simulink model "CM660A_HwTq1Meas"  (R2013b)
settings: Solver=FixedStepDiscrete  StartTime=0.0  StopTime=20  FixedStep=0.002  RelTol=1e-3
values from neighbouring files (symbols this model uses):
  ELECGLBPRM_HWTQOFFS_HWNWTMTR_F32 = DataDict.Constant    [CM660A_HwTq1Meas_DataDict.m]
  ELECGLBPRM_HWTQSATNLOWRLIM_HWNWTMTR_F32 = DataDict.Constant    [CM660A_HwTq1Meas_DataDict.m]
  ELECGLBPRM_HWTQSATNUPPRLIM_HWNWTMTR_F32 = DataDict.Constant    [CM660A_HwTq1Meas_DataDict.m]
  ELECGLBPRM_HWTQSCA_ULS_F32 = DataDict.Constant    [CM660A_HwTq1Meas_DataDict.m]
  ELECGLBPRM_NOFLT_CNT_U08 = DataDict.Constant    [CM660A_HwTq1Meas_DataDict.m]
  ELECGLBPRM_OFFSTRIMNOTPRFM_CNT_U08 = DataDict.Constant    [CM660A_HwTq1Meas_DataDict.m]
  ELECGLBPRM_PRTCLFLT_CNT_U08 = DataDict.Constant    [CM660A_HwTq1Meas_DataDict.m]
  ELECGLBPRM_SNSRINTFLT_CNT_U08 = DataDict.Constant    [CM660A_HwTq1Meas_DataDict.m]
  HwTq1MeasHwTq1PrtclFltFailStep = DataDict.Calibration    [CM660A_HwTq1Meas_DataDict.m]
  HwTq1MeasHwTq1PrtclFltPassStep = DataDict.Calibration    [CM660A_HwTq1Meas_DataDict.m]
  RACKLIMRCCWEOTSCA_ULS_F32 = DataDict.Constant    [CM660A_HwTq1Meas_DataDict.m]
  RACKLIMRCWEOTSCA_ULS_F32 = DataDict.Constant    [CM660A_HwTq1Meas_DataDict.m]
undefined symbols (not defined in the file or in its folder): NtcNr1, NtcSts1, sigbuilder_block, SigQlfr1
libraries: simulink x25, NxtrNvM x3, NxtrLim x2
(part 2 of 3)

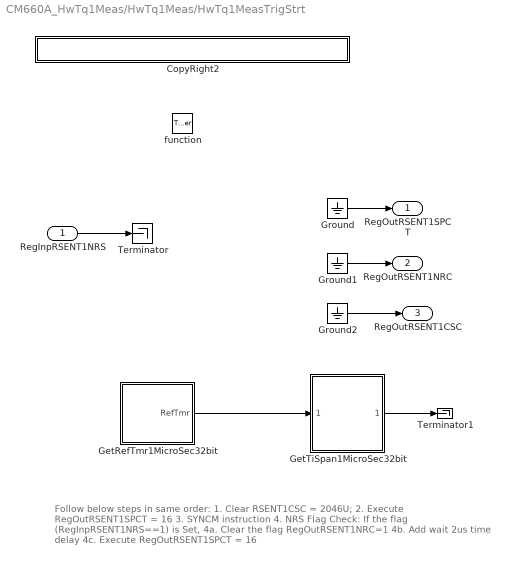
== system CM660A_HwTq1Meas/HwTq1Meas/HwTq1MeasTrigStrt ==
  note: Follow below steps in same order:
      |
      | 1. Clear RSENT1CSC = 2046U;
      | 2. Execute RegOutRSENT1SPCT = 16
      | 3. SYNCM instruction
      |
      | 4. NRS Flag Check: If the flag (RegInpRSENT1NRS==1) is Set,
      | 	4a. Clear the flag RegOutRSENT1NRC=1
      | 	4b. Add wait 2us time delay
      | 	4c. Execute RegOutRSENT1SPCT = 16
  RegInpRSENT1NRS : Inport
  function : TriggerPort  TriggerType=function-call
  CopyRight2 : Subsystem  Description=|  mask(Copyright Information){none=on}
      | Copyright info block.                                               
      |                                                                     
      | Place copyright information at the top of every subsystem in design.
      mask prompts: none "No parameters"
      mask help: Place copyright information at the top of every subsystem in design.
      mask Display:
      | NxtrConf = 'Nexteer Confidential';
      | 
      | sys = bdroot; %handle for the current model ("system")
      | first = get_param(sys,'Created');
      | first = first(end-3:end);  %year is last four digits
      | 
      | last = get_param(sys,'LastModifiedDate');
      | if isempty(last)
      |     last = datestr(now,'yyyy');
      | else
      |     last = last(end-3:end);
      | end
      | 
      | if strcmp(first,last)
      |     fprintf('%s -- Copyright %s Nexteer',NxtrConf,first)
      | else
      |     fprintf('%s -- %s%s- %s Nexteer',NxtrConf,char(169),first,last)
      | end
  GetRefTmr1MicroSec32bit : Subsystem
      settings: AttributesFormatString=Client Call : Start Time
  GetTiSpan1MicroSec32bit : Subsystem
  Ground : Ground
  Ground1 : Ground
  Ground2 : Ground
  Terminator : Terminator
  Terminator1 : Terminator
  RegOutRSENT1SPCT : Outport
  RegOutRSENT1NRC : Outport  Port=2
  RegOutRSENT1CSC : Outport  Port=3
  wires:
  ? -> ?
  Ground1/1 -> RegOutRSENT1NRC/1
  Ground/1 -> RegOutRSENT1SPCT/1
  Ground2/1 -> RegOutRSENT1CSC/1
  RegInpRSENT1NRS/1 -> Terminator/1
  GetTiSpan1MicroSec32bit/1(TiSpan) -> Terminator1/1
  GetRefTmr1MicroSec32bit/1(RefTmr) -> GetTiSpan1MicroSec32bit/1(RefTmr)

== system CM660A_HwTq1Meas/Simulated_Input1/CopyRight2 ==

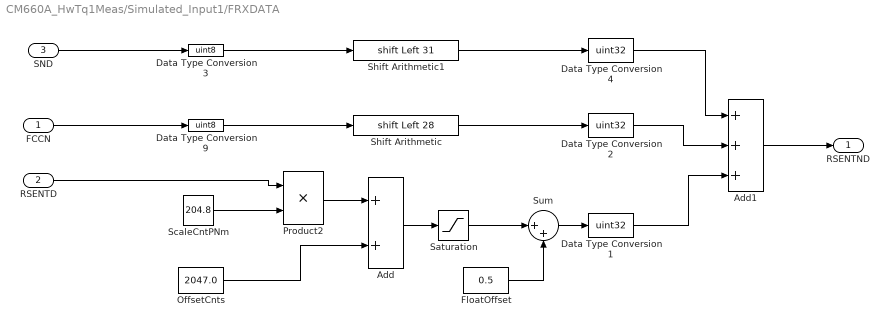
== system CM660A_HwTq1Meas/Simulated_Input1/FRXDATA ==
  FCCN : Inport
  RSENTD : Inport  Port=2
  SND : Inport  Port=3
  Add : Sum
  Add1 : Sum  Inputs=+++
  Data Type Conversion1 : DataTypeConversion  OutDataTypeStr=uint32
  Data Type Conversion2 : DataTypeConversion  OutDataTypeStr=uint32
  Data Type Conversion3 : DataTypeConversion  OutDataTypeStr=uint8
  Data Type Conversion4 : DataTypeConversion  OutDataTypeStr=uint32
  Data Type Conversion9 : DataTypeConversion  OutDataTypeStr=uint8
  FloatOffset : Constant  Value=0.5
  OffsetCnts : Constant  Value=2047.0
  Product2 : Product
  Saturation : Saturate  UpperLimit=4095.0  LowerLimit=0.0
  ScaleCntPNm : Constant  Value=204.8
  Shift Arithmetic : ArithShift  BitShiftNumber=28  BitShiftDirection=Left
  Shift Arithmetic1 : ArithShift  BitShiftNumber=31  BitShiftDirection=Left
  Sum : Sum  Inputs=|++
  RSENTND : Outport
  wires:
  Data Type Conversion4/1 -> Add1/1
  Shift Arithmetic1/1 -> Data Type Conversion4/1
  Data Type Conversion3/1 -> Shift Arithmetic1/1
  SND/1 -> Data Type Conversion3/1
  Data Type Conversion2/1 -> Add1/2
  Shift Arithmetic/1 -> Data Type Conversion2/1
  Add1/1 -> RSENTND/1
  Data Type Conversion1/1 -> Add1/3
  Data Type Conversion9/1 -> Shift Arithmetic/1
  FCCN/1 -> Data Type Conversion9/1
  Sum/1 -> Data Type Conversion1/1
  FloatOffset/1 -> Sum/2
  Saturation/1 -> Sum/1
  Add/1 -> Saturation/1
  OffsetCnts/1 -> Add/2
  Product2/1 -> Add/1
  ScaleCntPNm/1 -> Product2/2
  RSENTD/1 -> Product2/1

== system CM660A_HwTq1Meas/Simulated_Input1/FRXDATA1 ==
  Snsr0CS : Inport
  Snsr0FRS : Inport  Port=2
  Add1 : Sum
  Data Type Conversion1 : DataTypeConversion  OutDataTypeStr=uint32
  Data Type Conversion9 : DataTypeConversion  OutDataTypeStr=uint32
  Shift Arithmetic2 : ArithShift  BitShiftNumber=1  BitShiftDirection=Left
  RSENTCS : Outport
  wires:
  Shift Arithmetic2/1 -> Add1/1
  Data Type Conversion9/1 -> Shift Arithmetic2/1
  Data Type Conversion1/1 -> Add1/2
  Snsr0FRS/1 -> Data Type Conversion1/1
  Add1/1 -> RSENTCS/1
  Snsr0CS/1 -> Data Type Conversion9/1

== system CM660A_HwTq1Meas/Simulated_Input1/FRXDATA2 ==
  Snsr0IDD : Inport
  CW : Inport  Port=2
  CCW : Inport  Port=3
  Data Type Conversion2 : DataTypeConversion  OutDataTypeStr=uint32
  Display : Display
  Display1 : Display
  Display2 : Display
  RackLimrEotCal : MATLAB Function  TreatAsAtomicUnit=on
  RSENTSRXD : Outport
  wires:
  Data Type Conversion2/1 -> RackLimrEotCal/1(SensId)
  CCW/1 -> RackLimrEotCal/3(Ccw), Display2/1
  CW/1 -> RackLimrEotCal/2(Cw), Display/1
  Snsr0IDD/1 -> Data Type Conversion2/1
  RackLimrEotCal/1(RsentIdd) -> RSENTSRXD/1, Display1/1

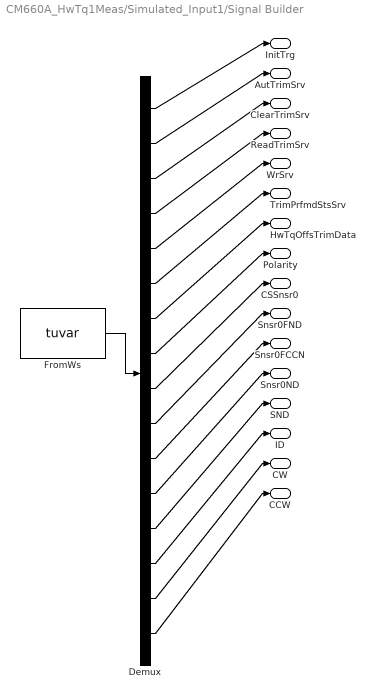
== system CM660A_HwTq1Meas/Simulated_Input1/Signal Builder ==
  Demux : Demux  Tag=STV Demux  Outputs=16
  FromWs : FromWorkspace  Tag=STV FromWs  VariableName=tuvar  SampleTime=0  OutputAfterFinalValue=Holding final value
      SigBuilderData=|
      | common.afterFinalStr = 'Hold final value'
      | common.sampleTime = '0'
      | dataSet(1).timeRange = [0 20]
      | dataSet(1).name = 'IdealSignal'
      | dataSet(2).timeRange = [0 20]
      | dataSet(2).name = 'Faults'
      | dataSet(3).timeRange = [0 20]
      | dataSet(3).name = 'Service'
      | sbobj.Groups(1).Name = 'IdealSignal'
      | sbobj.Groups(1).Signals(1).Name = 'InitTrg'
      | sbobj.Groups(1).Signals(1).XData = [0 0.02 0.02 0.06 0.06 20]
      | sbobj.Groups(1).Signals(1).YData = [0 0 1 1 0 0]
      | sbobj.Groups(1).Signals(2).Name = 'AutTrimSrv'
      | sbobj.Groups(1).Signals(2).XData = [0 20]
      | sbobj.Groups(1).Signals(2).YData = [0 0]
      | sbobj.Groups(1).Signals(3).Name = 'ClearTrimSrv'
      | sbobj.Groups(1).Signals(3).XData = [0 20]
      | sbobj.Groups(1).Signals(3).YData = [0 0]
      | sbobj.Groups(1).Signals(4).Name = 'ReadTrimSrv'
      | sbobj.Groups(1).Signals(4).XData = [0 20]
      | sbobj.Groups(1).Signals(4).YData = [0 0]
      | sbobj.Groups(1).Signals(5).Name = 'WrSrv'
      | sbobj.Groups(1).Signals(5).XData = [0 0.04 0.04 0.08 0.08 20]
      | sbobj.Groups(1).Signals(5).YData = [0 0 1 1 0 0]
      | sbobj.Groups(1).Signals(6).Name = 'TrimPrfmdStsSrv'
      | sbobj.Groups(1).Signals(6).XData = [0 20]
      | sbobj.Groups(1).Signals(6).YData = [0 0]
      | sbobj.Groups(1).Signals(7).Name = 'HwTqOffsTrimData'
      | sbobj.Groups(1).Signals(7).XData = [0 20]
      | sbobj.Groups(1).Signals(7).YData = [0 0]
      | sbobj.Groups(1).Signals(8).Name = 'Polarity'
      | sbobj.Groups(1).Signals(8).XData = [0 20]
      | sbobj.Groups(1).Signals(8).YData = [1 1]
      | sbobj.Groups(1).Signals(9).Name = 'CSSnsr0'
      | sbobj.Groups(1).Signals(9).XData = [0 20]
      | sbobj.Groups(1).Signals(9).YData = [0 0]
      | sbobj.Groups(1).Signals(10).Name = 'Snsr0FND'
      | sbobj.Groups(1).Signals(10).XData = [0 20]
      | sbobj.Groups(1).Signals(10).YData = [1 1]
      | sbobj.Groups(1).Signals(11).Name = 'Snsr0FCCN'
      | sbobj.Groups(1).Signals(11).XData = [0 20]
      | sbobj.Groups(1).Signals(11).YData = [0 0]
      | sbobj.Groups(1).Signals(12).Name = 'Snsr0ND'
      | sbobj.Groups(1).Signals(12).XData = [0 2 2 4 4 6 6 8 8 10 10 12 12 14 14 16 16 18 18 20]
      | sbobj.Groups(1).Signals(12).YData = [-10 10 -10 10 -10 10 -10 10 -10 10 -10 10 -10 10 -10 10 -10 10 -10 10]
      | sbobj.Groups(1).Signals(13).Name = 'SND'
      | sbobj.Groups(1).Signals(13).XData = [0 0.1 0.1 0.2 0.2 0.3 0.3 0.4 0.4 0.5 0.5 0.6 0.6 0.7 0.7 0.8 0.8 0.9 0.9 1 1 1.1 1.1 1.2 1.2 1.3 1.3 1.4 1.4 1.5 1.5 1.6 1.6 1.7 1.7 1.8 1.8 1.9 1.9 2 2 2.1 2.1 2.2 2.2 2.3 2.3 2.4 2.4 2.5 2.5 2.6 2.6 2.7 2.7 2.8 2.8 2.9 2.9 3 3 3.1 3.1 3.2 3.2 3.3 3.3 3.4 3.4 3.5 3.5 3.6 3.6 3.7 3.7 3.8 3.8 3.9 3.9 4 4 4.1 4.1 4.2 4.2 4.3 4.3 4.4 4.4 4.5 4.5 4.6 4.6 4.7 4.7 4.8 4.8 4.9 4.9 5 5 5.1 5.1 5.2 5.2 5.3 5.3 5.4 5.4 5.5 5.5 5.6 5.6 5.7 5.7 5.8 5.8 5.9 5.9 6 6 6.1 6.1 6.2 6.2 6.3 6.3 6.4 6.4 6.5 6.5 6.6 6.6 6.7 6.7 6.8 6.8 6.9 6.9 7 7 7.1 7.1 7.2 7.2 7.3 7.3 7.4 7.4 7.5 7.5 7.6 7.6 7.7 7.7 7.8 7.8 7.9 7.9 8 8 8.1 8.1 8.2 8.2 8.3 8.3 8.4 8.4 8.5 8.5 8.6 8.6 8.7 8.7 8.8 8.8 8.9 8.9 9 9 9.1 9.1 9.2 9.2 9.3 9.3 9.4 9.4 9.5 9.5 9.6 9.6 9.7 9.7 9.8 9.8 9.9 9.9 10 10 10.1 10.1 10.2 10.2 10.3 10.3 10.4 10.4 10.5 10.5 10.6 10.6 10.7 10.7 10.8 10.8 10.9 10.9 11 11 11.1 11.1 11.2 11.2 11.3 11.3 11.4 11.4 11.5 11.5 11.6 11.6 11.7 11.7 11.8 11.8 11.9 11.9 12 12 12.1 12.1 12.2 12.2 12.3 12.3 12.4 12.4 12.5 12.5 12.6 12.6 12.7 12.7 12.8 12.8 12.9 12.9 13 13 13.1 13.1 13.2 13.2 13.3 13.3 13.4 13.4 13.5 13.5 13.6 13.6 13.7 13.7 13.8 13.8 13.9 13.9 14 14 14.1 14.1 14.2 14.2 14.3 14.3 14.4 14.4 14.5 14.5 14.6 14.6 14.7 14.7 14.8 14.8 14.9 14.9 15 15 15.1 15.1 15.2 15.2 15.3 15.3 15.4 15.4 15.5 15.5 15.6 15.6 15.7 15.7 15.8 15.8 15.9 15.9 16 16 16.1 16.1 16.2 16.2 16.3 16.3 16.4 16.4 16.5 16.5 16.6 16.6 16.7 16.7 16.8 16.8 16.9 16.9 17 17 17.1 17.1 17.2 17.2 17.3 17.3 17.4 17.4 17.5 17.5 17.6 17.6 17.7 17.7 17.8 17.8 17.9 17.9 18 18 18.1 18.1 18.2 18.2 18.3 18.3 18.4 18.4 18.5 18.5 18.6 18.6 18.7 18.7 18.8 18.8 18.9 18.9 19 19 19.1 19.1 19.2 19.2 19.3 19.3 19.4 19.4 19.5 19.5 19.6 19.6 19.7 19.7 19.8 19.8 19.9 19.9 20]
      | sbobj.Groups(1).Signals(13).YData = [1 1 0 0 1 1 0 0 1 1 0 0 1 1 0 0 1 1 0 0 1 1 0 0 1 1 0 0 1 1 0 0 1 1 0 0 1 1 0 0 1 1 0 0 1 1 0 0 1 1 0 0 1 1 0 0 1 1 0 0 1 1 0 0 1 1 0 0 1 1 0 0 1 1 0 0 1 1 0 0 1 1 0 0 1 1 0 0 1 1 0 0 1 1 0 0 1 1 0 0 1 1 0 0 1 1 0 0 1 1 0 0 1 1 0 0 1 1 0 0 1 1 0 0 1 1 0 0 1 1 0 0 1 1 0 0 1 1 0 0 1 1 0 0 1 1 0 0 1 1 0 0 1 1 0 0 1 1 0 0 1 1 0 0 1 1 0 0 1 1 0 0 1 1 0 0 1 1 0 0 1 1 0 0 1 1 0 0 1 1 0 0 1 1 0 0 1 1 0 0 1 1 0 0 1 1 0 0 1 1 0 0 1 1 0 0 1 1 0 0 1 1 0 0 1 1 0 0 1 1 0 0 1 1 0 0 1 1 0 0 1 1 0 0 1 1 0 0 1 1 0 0 1 1 0 0 1 1 0 0 1 1 0 0 1 1 0 0 1 1 0 0 1 1 0 0 1 1 0 0 1 1 0 0 1 1 0 0 1 1 0 0 1 1 0 0 1 1 0 0 1 1 0 0 1 1 0 0 1 1 0 0 1 1 0 0 1 1 0 0 1 1 0 0 1 1 0 0 1 1 0 0 1 1 0 0 1 1 0 0 1 1 0 0 1 1 0 0 1 1 0 0 1 1 0 0 1 1 0 0 1 1 0 0 1 1 0 0 1 1 0 0 1 1 0 0 1 1 0 0 1 1 0 0 1 1 0 0 1 1 0 0 1 1 0 0 1 1 0 0]
      | sbobj.Groups(1).Signals(14).Name = 'ID'
      | sbobj.Groups(1).Signals(14).XData = [0 0.166666666667 0.166666666667 0.333333333333 0.333333333333 0.5 0.5 0.666666666667 0.666666666667 0.833333333333 0.833333333333 1 ... (240 elements, 1x240)]
      | sbobj.Groups(1).Signals(14).YData = [1 1 0 0 1 1 0 0 3 3 0 0 2 2 0 0 4 4 0 0 1 1 0 0 1 1 0 0 1 1 0 0 1 1 0 0 1 1 0 0 1 1 0 0 1 1 0 0 1 1 0 0 1 1 0 0 1 1 0 0 1 1 0 0 1 1 0 0 1 1 0 0 1 1 0 0 1 1 0 0 1 1 0 0 1 1 0 0 1 1 0 0 1 1 0 0 1 1 0 0 1 1 0 0 1 1 0 0 1 1 0 0 1 1 0 0 1 1 0 0 1 1 0 0 1 1 0 0 2 2 0 0 3 3 0 0 4 4 0 0 1 1 0 0 1 1 0 0 1 1 0 0 1 1 0 0 1 1 0 0 1 1 0 0 1 1 0 0 1 1 0 0 1 1 0 0 1 1 0 0 1 1 0 0 1 1 0 0 1 1 0 0 1 1 0 0 1 1 0 0 1 1 0 0 1 1 0 0 1 1 0 0 1 1 0 0 1 1 0 0 1 1 0 0 1 1 0 0 1 1 0 0 1 1 0 0 1 1 0 0]
      | sbobj.Groups(1).Signals(15).Name = 'CW'
      | sbobj.Groups(1).Signals(15).XData = [0 5 5 10 10 15 15 20]
      | sbobj.Groups(1).Signals(15).YData = [600 600 0 0 500 500 100 100]
      | sbobj.Groups(1).Signals(16).Name = 'CCW'
      | sbobj.Groups(1).Signals(16).XData = [0 5 5 10 10 15 15 20]
      | sbobj.Groups(1).Signals(16).YData = [500 500 200 200 650 650 201 201]
      | sbobj.Groups(1).TimeRange = [0 20]
      | sbobj.Groups(2).Name = 'Faults'
      | sbobj.Groups(2).Signals(1).Name = 'InitTrg'
      | sbobj.Groups(2).Signals(1).XData = [0 0.02 0.02 0.06 0.06 20]
      | sbobj.Groups(2).Signals(1).YData = [0 0 1 1 0 0]
      | sbobj.Groups(2).Signals(2).Name = 'AutTrimSrv'
      | sbobj.Groups(2).Signals(2).XData = [0 20]
      | sbobj.Groups(2).Signals(2).YData = [0 0]
      | sbobj.Groups(2).Signals(3).Name = 'ClearTrimSrv'
      | sbobj.Groups(2).Signals(3).XData = [0 20]
      | sbobj.Groups(2).Signals(3).YData = [0 0]
      | sbobj.Groups(2).Signals(4).Name = 'ReadTrimSrv'
      | sbobj.Groups(2).Signals(4).XData = [0 20]
      | sbobj.Groups(2).Signals(4).YData = [0 0]
      | sbobj.Groups(2).Signals(5).Name = 'WrSrv'
      | sbobj.Groups(2).Signals(5).XData = [0 0.06 0.06 0.12 0.12 20]
      | sbobj.Groups(2).Signals(5).YData = [0 0 1 1 0 0]
      | sbobj.Groups(2).Signals(6).Name = 'TrimPrfmdStsSrv'
      | sbobj.Groups(2).Signals(6).XData = [0 20]
      | sbobj.Groups(2).Signals(6).YData = [0 0]
      | sbobj.Groups(2).Signals(7).Name = 'HwTqOffsTrimData'
      | sbobj.Groups(2).Signals(7).XData = [0 20]
      | sbobj.Groups(2).Signals(7).YData = [0 0]
      | sbobj.Groups(2).Signals(8).Name = 'Polarity'
      | sbobj.Groups(2).Signals(8).XData = [0 11 11 20]
      | sbobj.Groups(2).Signals(8).YData = [-1 -1 1 1]
      | sbobj.Groups(2).Signals(9).Name = 'CSSnsr0'
      | sbobj.Groups(2).Signals(9).XData = [0 2.54 2.54 2.88 2.88 20]
      | sbobj.Groups(2).Signals(9).YData = [0 0 2 2 0 0]
      | sbobj.Groups(2).Signals(10).Name = 'Snsr0FND'
      | sbobj.Groups(2).Signals(10).XData = [0 14.54 14.54 14.78 14.78 20]
      | sbobj.Groups(2).Signals(10).YData = [1 1 0 0 1 1]
      | sbobj.Groups(2).Signals(11).Name = 'Snsr0FCCN'
      | sbobj.Groups(2).Signals(11).XData = [0 12.02 12.02 12.26 12.26 20]
      | sbobj.Groups(2).Signals(11).YData = [0 0 1 1 0 0]
      | sbobj.Groups(2).Signals(12).Name = 'Snsr0ND'
      | sbobj.Groups(2).Signals(12).XData = [0 2 2 4 4 6 6 8 8 10 10 12 12 14 14 16 16 18 18 20]
      | sbobj.Groups(2).Signals(12).YData = [-10 10 -10 10 -10 10 -10 10 -10 10 -10 10 -10 10 -10 10 -10 10 -10 10]
      | sbobj.Groups(2).Signals(13).Name = 'SND'
      | sbobj.Groups(2).Signals(13).XData = [0 0.1 0.1 0.2 0.2 0.3 0.3 0.4 0.4 0.5 0.5 0.6 0.6 0.7 0.7 0.8 0.8 0.9 0.9 1 1 1.1 1.1 1.2 1.2 1.3 1.3 1.4 1.4 1.5 1.5 1.6 1.6 1.7 1.7 1.8 1.8 1.9 1.9 2 2 2.1 2.1 2.2 2.2 2.3 2.3 2.4 2.4 2.5 2.5 2.6 2.6 2.7 2.7 2.8 2.8 2.9 2.9 3 3 3.1 3.1 3.2 3.2 3.3 3.3 3.4 3.4 3.5 3.5 3.6 3.6 3.7 3.7 3.8 3.8 3.9 3.9 4 4 4.1 4.1 4.2 4.2 4.3 4.3 4.4 4.4 4.5 4.5 4.6 4.6 4.7 4.7 4.8 4.8 4.9 4.9 5 5 5.1 5.1 5.2 5.2 5.3 5.3 5.4 5.4 5.5 5.5 5.6 5.6 5.7 5.7 5.8 5.8 5.9 5.9 6 6 6.1 6.1 6.2 6.2 6.3 6.3 6.4 6.4 6.5 6.5 6.6 6.6 6.7 6.7 6.8 6.8 6.9 6.9 7 7 7.1 7.1 7.2 7.2 7.3 7.3 7.4 7.4 7.5 7.5 7.6 7.6 7.7 7.7 7.8 7.8 7.9 7.9 8 8 8.1 8.1 8.2 8.2 8.3 8.3 8.4 8.4 8.5 8.5 8.6 8.6 8.7 8.7 8.8 8.8 8.9 8.9 9 9 9.1 9.1 9.2 9.2 9.3 9.3 9.4 9.4 9.5 9.5 9.6 9.6 9.7 9.7 9.8 9.8 9.9 9.9 10 10 10.1 10.1 10.2 10.2 10.3 10.3 10.4 10.4 10.5 10.5 10.6 10.6 10.7 10.7 10.8 10.8 10.9 10.9 11 11 11.1 11.1 11.2 11.2 11.3 11.3 11.4 11.4 11.5 11.5 11.6 11.6 11.7 11.7 11.8 11.8 11.9 11.9 12 12 12.1 12.1 12.2 12.2 12.3 12.3 12.4 12.4 12.5 12.5 12.6 12.6 12.7 12.7 12.8 12.8 12.9 12.9 13 13 13.1 13.1 13.2 13.2 13.3 13.3 13.4 13.4 13.5 13.5 13.6 13.6 13.7 13.7 13.8 13.8 13.9 13.9 14 14 14.1 14.1 14.2 14.2 14.3 14.3 14.4 14.4 14.5 14.5 14.6 14.6 14.7 14.7 14.8 14.8 14.9 14.9 15 15 15.1 15.1 15.2 15.2 15.3 15.3 15.4 15.4 15.5 15.5 15.6 15.6 15.7 15.7 15.8 15.8 15.9 15.9 16 16 16.1 16.1 16.2 16.2 16.3 16.3 16.4 16.4 16.5 16.5 16.6 16.6 16.7 16.7 16.8 16.8 16.9 16.9 17 17 17.1 17.1 17.2 17.2 17.3 17.3 17.4 17.4 17.5 17.5 17.6 17.6 17.7 17.7 17.8 17.8 17.9 17.9 18 18 18.1 18.1 18.2 18.2 18.3 18.3 18.4 18.4 18.5 18.5 18.6 18.6 18.7 18.7 18.8 18.8 18.9 18.9 19 19 19.1 19.1 19.2 19.2 19.3 19.3 19.4 19.4 19.5 19.5 19.6 19.6 19.7 19.7 19.8 19.8 19.9 19.9 20]
      | sbobj.Groups(2).Signals(13).YData = [1 1 0 0 1 1 0 0 1 1 0 0 1 1 0 0 1 1 0 0 1 1 0 0 1 1 0 0 1 1 0 0 1 1 0 0 1 1 0 0 1 1 0 0 1 1 0 0 1 1 0 0 1 1 0 0 1 1 0 0 1 1 0 0 1 1 0 0 1 1 0 0 1 1 0 0 1 1 0 0 1 1 0 0 1 1 0 0 1 1 0 0 1 1 0 0 1 1 0 0 1 1 0 0 1 1 0 0 1 1 0 0 1 1 0 0 1 1 0 0 1 1 0 0 1 1 0 0 1 1 0 0 1 1 0 0 1 1 0 0 1 1 0 0 1 1 0 0 1 1 0 0 1 1 0 0 1 1 0 0 1 1 0 0 1 1 0 0 1 1 0 0 1 1 0 0 1 1 0 0 1 1 0 0 1 1 0 0 1 1 0 0 1 1 0 0 1 1 0 0 1 1 0 0 1 1 0 0 1 1 0 0 1 1 0 0 1 1 0 0 1 1 0 0 1 1 0 0 1 1 0 0 1 1 0 0 1 1 0 0 1 1 0 0 1 1 0 0 1 1 0 0 1 1 0 0 1 1 0 0 1 1 0 0 1 1 0 0 1 1 0 0 1 1 0 0 1 1 0 0 1 1 0 0 1 1 0 0 1 1 0 0 1 1 0 0 1 1 0 0 1 1 0 0 1 1 0 0 1 1 0 0 1 1 0 0 1 1 0 0 1 1 0 0 1 1 0 0 1 1 0 0 1 1 0 0 1 1 0 0 1 1 0 0 1 1 0 0 1 1 0 0 1 1 0 0 1 1 0 0 1 1 0 0 1 1 0 0 1 1 0 0 1 1 0 0 1 1 0 0 1 1 0 0 1 1 0 0 1 1 0 0 1 1 0 0 1 1 0 0]
      | sbobj.Groups(2).Signals(14).Name = 'ID'
      | sbobj.Groups(2).Signals(14).XData = [0 0.166666666667 0.166666666667 0.333333333333 0.333333333333 0.5 0.5 0.666666666667 0.666666666667 0.833333333333 0.833333333333 1 ... (238 elements, 1x238)]
      | sbobj.Groups(2).Signals(14).YData = [1 1 0 0 1 1 0 0 3 3 0 0 2 2 0 0 0 0 1 1 0 0 1 1 0 0 1 1 0 0 1 1 0 0 1 1 0 0 1 1 0 0 1 1 0 0 1 1 0 0 1 1 0 0 1 1 0 0 1 1 0 0 1 1 0 0 1 1 0 0 1 1 0 0 1 1 0 0 1 1 0 0 1 1 0 0 1 1 0 0 1 1 0 0 1 1 0 0 1 1 0 0 1 1 0 0 1 1 0 0 1 1 0 0 1 1 0 0 1 1 0 0 1 1 0 0 1 1 0 0 1 1 0 0 1 1 0 0 1 1 0 0 1 1 0 0 1 1 0 0 1 1 0 0 1 1 0 0 1 1 0 0 1 1 0 0 1 1 0 0 1 1 0 0 1 1 0 0 1 1 0 0 1 1 0 0 1 1 0 0 1 1 0 0 1 1 0 0 1 1 0 0 1 1 0 0 1 1 0 0 1 1 0 0 1 1 0 0 1 1 0 0 1 1 0 0 1 1 0 0 1 1 0 0 1 1 0 0]
      | sbobj.Groups(2).Signals(15).Name = 'CW'
      | sbobj.Groups(2).Signals(15).XData = [0 5 5 10 10 15 15 20]
      | sbobj.Groups(2).Signals(15).YData = [600.2 600.2 0 0 500 500 100 100]
      | sbobj.Groups(2).Signals(16).Name = 'CCW'
      | sbobj.Groups(2).Signals(16).XData = [0 5 5 10 10 15 15 20]
      | sbobj.Groups(2).Signals(16).YData = [500 500 200 200 650 650 201 201]
      | sbobj.Groups(2).TimeRange = [0 20]
      | sbobj.Groups(3).Name = 'Service'
      | sbobj.Groups(3).Signals(1).Name = 'InitTrg'
      | sbobj.Groups(3).Signals(1).XData = [0 0.02 0.02 0.06 0.06 20]
      | sbobj.Groups(3).Signals(1).YData = [0 0 1 1 0 0]
      | sbobj.Groups(3).Signals(2).Name = 'AutTrimSrv'
      | sbobj.Groups(3).Signals(2).XData = [0 0.58 0.58 0.68 0.68 16 16 16.1 16.1 20]
      | sbobj.Groups(3).Signals(2).YData = [0 0 1 1 0 0 1 1 0 0]
      | sbobj.Groups(3).Signals(3).Name = 'ClearTrimSrv'
      | sbobj.Groups(3).Signals(3).XData = [0 0.34 4.1 4.1 4.16 4.16 9.98 9.98 10.06 10.06 20]
      | sbobj.Groups(3).Signals(3).YData = [0 0 0 1 1 0 0 1 1 0 0]
      | sbobj.Groups(3).Signals(4).Name = 'ReadTrimSrv'
      | sbobj.Groups(3).Signals(4).XData = [0 1.24 1.24 1.32 1.32 4.62 4.62 4.7 4.7 6.84 6.84 6.92 6.92 10.38 10.38 10.46 10.46 16.72 16.72 16.8 16.8 20]
      | sbobj.Groups(3).Signals(4).YData = [0 0 1 1 0 0 1 1 0 0 1 1 0 0 1 1 0 0 1 1 0 0]
      | sbobj.Groups(3).Signals(5).Name = 'WrSrv'
      | sbobj.Groups(3).Signals(5).XData = [0 6.22 6.22 6.3 6.3 20]
      | sbobj.Groups(3).Signals(5).YData = [0 0 1 1 0 0]
      | sbobj.Groups(3).Signals(6).Name = 'TrimPrfmdStsSrv'
      | sbobj.Groups(3).Signals(6).XData = [0 1.24 1.24 1.32 1.32 4.64 4.64 4.7 4.7 6.84 6.84 6.92 6.92 10.64 10.64 10.72 10.72 16.74 16.74 16.82 16.82 20]
      | sbobj.Groups(3).Signals(6).YData = [0 0 1 1 0 0 1 1 0 0 1 1 0 0 1 1 0 0 1 1 0 0]
      | sbobj.Groups(3).Signals(7).Name = 'HwTqOffsTrimData'
      | sbobj.Groups(3).Signals(7).XData = [0 0.4 5.78 5.78 7.62 7.62 20]
      | sbobj.Groups(3).Signals(7).YData = [0 0 0 5 5 0 0]
      | sbobj.Groups(3).Signals(8).Name = 'Polarity'
      | sbobj.Groups(3).Signals(8).XData = [0 20]
      | sbobj.Groups(3).Signals(8).YData = [1 1]
      | sbobj.Groups(3).Signals(9).Name = 'CSSnsr0'
      | sbobj.Groups(3).Signals(9).XData = [0 20]
      | sbobj.Groups(3).Signals(9).YData = [0 0]
      | sbobj.Groups(3).Signals(10).Name = 'Snsr0FND'
      | sbobj.Groups(3).Signals(10).XData = [0 20]
      | sbobj.Groups(3).Signals(10).YData = [1 1]
      | sbobj.Groups(3).Signals(11).Name = 'Snsr0FCCN'
      | sbobj.Groups(3).Signals(11).XData = [0 20]
      | sbobj.Groups(3).Signals(11).YData = [0 0]
      | sbobj.Groups(3).Signals(12).Name = 'Snsr0ND'
      | sbobj.Groups(3).Signals(12).XData = [0 2 2 4 4 6 6 8 8 10 10 12 12 14 14 16 16 18 18 20]
      | sbobj.Groups(3).Signals(12).YData = [-10 10 -10 10 -10 10 -10 10 -10 10 -10 10 -10 10 -10 10 -10 10 -10 10]
      | sbobj.Groups(3).Signals(13).Name = 'SND'
      | sbobj.Groups(3).Signals(13).XData = [0 0.1 0.1 0.2 0.2 0.3 0.3 0.4 0.4 0.5 0.5 0.6 0.6 0.7 0.7 0.8 0.8 0.9 0.9 1 1 1.1 1.1 1.2 1.3 1.4 1.5 1.6 1.7 1.8 1.8 1.9 1.9 2 2 2.1 2.1 2.2 2.2 2.3 2.3 2.4 2.4 2.5 2.5 2.6 2.6 2.7 2.7 2.8 2.8 2.9 2.9 3 3 3.1 3.1 3.2 3.2 3.3 3.3 3.4 3.4 3.5 3.5 3.6 3.6 3.7 3.7 3.8 3.8 3.9 3.9 4 4 4.1 4.1 4.2 4.2 4.3 4.3 4.4 4.4 4.5 4.5 4.6 4.6 4.7 4.7 4.8 4.8 4.9 4.9 5 5 5.1 5.1 5.2 5.2 5.3 5.3 5.4 5.4 5.5 5.5 5.6 5.6 5.7 5.7 5.8 5.8 5.9 5.9 6 6 6.1 6.1 6.2 6.2 6.3 6.3 6.4 6.4 6.5 6.5 6.6 6.6 6.7 6.7 6.8 6.8 6.9 6.9 7 7 7.1 7.1 7.2 7.2 7.3 7.3 7.4 7.4 7.5 7.5 7.6 7.6 7.7 7.7 7.8 7.8 7.9 7.9 8 8 8.1 8.1 8.2 8.2 8.3 8.3 8.4 8.4 8.5 8.5 8.6 8.6 8.7 8.7 8.8 8.8 8.9 8.9 9 9 9.1 9.1 9.2 9.2 9.3 9.3 9.4 9.4 9.5 9.5 9.6 9.6 9.7 9.7 9.8 9.8 9.9 9.9 10 10 10.1 10.1 10.2 10.2 10.3 10.3 10.4 10.4 10.5 10.5 10.6 10.6 10.7 10.7 10.8 10.8 10.9 10.9 11 11 11.1 11.1 11.2 11.2 11.3 11.3 11.4 11.4 11.5 11.5 11.6 11.6 11.7 11.7 11.8 11.8 11.9 11.9 12 12 12.1 12.1 12.2 12.2 12.3 12.3 12.4 12.4 12.5 12.5 12.6 12.6 12.7 12.7 12.8 12.8 12.9 12.9 13 13 13.1 13.1 13.2 13.2 13.3 13.3 13.4 13.4 13.5 13.5 13.6 13.6 13.7 13.7 13.8 13.8 13.9 13.9 14 14 14.1 14.1 14.2 14.2 14.3 14.3 14.4 14.4 14.5 14.5 14.6 14.6 14.7 14.7 14.8 14.8 14.9 14.9 15 15 15.1 15.1 15.2 15.2 15.3 15.3 15.4 15.4 15.5 15.5 15.6 15.6 15.7 15.7 15.8 15.8 15.9 15.9 16 16 16.1 16.1 16.2 16.2 16.3 16.3 16.4 16.4 16.5 16.5 16.6 16.6 16.7 16.7 16.8 16.8 16.9 16.9 17 17 17.1 17.1 17.2 17.2 17.3 17.3 17.4 17.4 17.5 17.5 17.6 17.6 17.7 17.7 17.8 17.8 17.9 17.9 18 18 18.1 18.1 18.2 18.2 18.3 18.3 18.4 18.4 18.5 18.5 18.6 18.6 18.7 18.7 18.8 18.8 18.9 18.9 19 19 19.1 19.1 19.2 19.2 19.3 19.3 19.4 19.4 19.5 19.5 19.6 19.6 19.7 19.7 19.8 19.8 19.9 19.9 20]
      | sbobj.Groups(3).Signals(13).YData = [1 1 0 0 1 1 0 0 1 1 0 0 1 1 0 0 1 1 0 0 1 1 0 0 0 0 0 0 0 0 1 1 0 0 1 1 0 0 1 1 0 0 1 1 0 0 1 1 0 0 1 1 0 0 1 1 0 0 1 1 0 0 1 1 0 0 1 1 0 0 1 1 0 0 1 1 0 0 1 1 0 0 1 1 0 0 1 1 0 0 1 1 0 0 1 1 0 0 1 1 0 0 1 1 0 0 1 1 0 0 1 1 0 0 1 1 0 0 1 1 0 0 1 1 0 0 1 1 0 0 1 1 0 0 1 1 0 0 1 1 0 0 1 1 0 0 1 1 0 0 1 1 0 0 1 1 0 0 1 1 0 0 1 1 0 0 1 1 0 0 1 1 0 0 1 1 0 0 1 1 0 0 1 1 0 0 1 1 0 0 1 1 0 0 1 1 0 0 1 1 0 0 1 1 0 0 1 1 0 0 1 1 0 0 1 1 0 0 1 1 0 0 1 1 0 0 1 1 0 0 1 1 0 0 1 1 0 0 1 1 0 0 1 1 0 0 1 1 0 0 1 1 0 0 1 1 0 0 1 1 0 0 1 1 0 0 1 1 0 0 1 1 0 0 1 1 0 0 1 1 0 0 1 1 0 0 1 1 0 0 1 1 0 0 1 1 0 0 1 1 0 0 1 1 0 0 1 1 0 0 1 1 0 0 1 1 0 0 1 1 0 0 1 1 0 0 1 1 0 0 1 1 0 0 1 1 0 0 1 1 0 0 1 1 0 0 1 1 0 0 1 1 0 0 1 1 0 0 1 1 0 0 1 1 0 0 1 1 0 0 1 1 0 0 1 1 0 0 1 1 0 0 1 1 0 0 1 1 0 0 1 1 0 0]
      | sbobj.Groups(3).Signals(14).Name = 'ID'
      | sbobj.Groups(3).Signals(14).XData = [0 0.166666666667 0.166666666667 0.333333333333 0.333333333333 0.5 0.5 0.666666666667 0.666666666667 0.833333333333 0.833333333333 1 ... (240 elements, 1x240)]
      | sbobj.Groups(3).Signals(14).YData = [1 1 0 0 1 1 0 0 3 3 0 0 2 2 0 0 4 4 0 0 1 1 0 0 1 1 0 0 1 1 0 0 1 1 0 0 1 1 0 0 1 1 0 0 1 1 0 0 1 1 0 0 1 1 0 0 1 1 0 0 1 1 0 0 1 1 0 0 1 1 0 0 1 1 0 0 1 1 0 0 1 1 0 0 1 1 0 0 1 1 0 0 1 1 0 0 1 1 0 0 1 1 0 0 1 1 0 0 1 1 0 0 1 1 0 0 1 1 0 0 1 1 0 0 1 1 0 0 1 1 0 0 1 1 0 0 1 1 0 0 1 1 0 0 1 1 0 0 1 1 0 0 1 1 0 0 1 1 0 0 1 1 0 0 1 1 0 0 1 1 0 0 1 1 0 0 1 1 0 0 1 1 0 0 1 1 0 0 1 1 0 0 1 1 0 0 1 1 0 0 1 1 0 0 1 1 0 0 1 1 0 0 1 1 0 0 1 1 0 0 1 1 0 0 1 1 0 0 1 1 0 0 1 1 0 0 1 1 0 0]
      | sbobj.Groups(3).Signals(15).Name = 'CW'
      | sbobj.Groups(3).Signals(15).XData = [0 5 5 10 10 15 15 20]
      | sbobj.Groups(3).Signals(15).YData = [600.2 600.2 0 0 500 500 100 100]
      | sbobj.Groups(3).Signals(16).Name = 'CCW'
      | sbobj.Groups(3).Signals(16).XData = [0 5 5 10 10 15 15 20]
      | sbobj.Groups(3).Signals(16).YData = [500 500 200 200 650 650 201 201]
      | sbobj.Groups(3).TimeRange = [0 20]
  InitTrg : Outport  Tag=STV Outport
  AutTrimSrv : Outport  Tag=STV Outport  Port=2
  ClearTrimSrv : Outport  Tag=STV Outport  Port=3
  ReadTrimSrv : Outport  Tag=STV Outport  Port=4
  WrSrv : Outport  Tag=STV Outport  Port=5
  TrimPrfmdStsSrv : Outport  Tag=STV Outport  Port=6
  HwTqOffsTrimData : Outport  Tag=STV Outport  Port=7
  Polarity : Outport  Tag=STV Outport  Port=8
  CSSnsr0 : Outport  Tag=STV Outport  Port=9
  Snsr0FND : Outport  Tag=STV Outport  Port=10
  Snsr0FCCN : Outport  Tag=STV Outport  Port=11
  Snsr0ND : Outport  Tag=STV Outport  Port=12
  SND : Outport  Tag=STV Outport  Port=13
  ID : Outport  Tag=STV Outport  Port=14
  CW : Outport  Tag=STV Outport  Port=15
  CCW : Outport  Tag=STV Outport  Port=16
  wires:
  Demux/16 -> CCW/1
  Demux/15 -> CW/1
  Demux/14 -> ID/1
  Demux/13 -> SND/1
  Demux/12 -> Snsr0ND/1
  Demux/11 -> Snsr0FCCN/1
  Demux/10 -> Snsr0FND/1
  Demux/9 -> CSSnsr0/1
  Demux/8 -> Polarity/1
  Demux/7 -> HwTqOffsTrimData/1
  Demux/6 -> TrimPrfmdStsSrv/1
  Demux/5 -> WrSrv/1
  Demux/4 -> ReadTrimSrv/1
  Demux/3 -> ClearTrimSrv/1
  Demux/2 -> AutTrimSrv/1
  Demux/1 -> InitTrg/1
  FromWs/1 -> Demux/1

== system CM660A_HwTq1Meas/HwTq1Meas/HwTq1MeasHwTq1AutTrim/CopyRight2 ==

== system CM660A_HwTq1Meas/HwTq1Meas/HwTq1MeasHwTq1ClrTrim/CopyRight2 ==

== system CM660A_HwTq1Meas/HwTq1Meas/HwTq1MeasHwTq1ReadTrim/CopyRight2 ==

== system CM660A_HwTq1Meas/HwTq1Meas/HwTq1MeasHwTq1TrimPrfmdSts/CopyRight2 ==

== system CM660A_HwTq1Meas/HwTq1Meas/HwTq1MeasHwTq1WrTrim/CopyRight2 ==

== system CM660A_HwTq1Meas/HwTq1Meas/HwTq1MeasInit1/CopyRight2 ==

== system CM660A_HwTq1Meas/HwTq1Meas/HwTq1MeasInit1/GetRefTmr1MicroSec32bit ==
  CopyRight2 : Subsystem  Description=|  mask(Copyright Information){none=on}
      | Copyright info block.                                               
      |                                                                     
      | Place copyright information at the top of every subsystem in design.
      mask prompts: none "No parameters"
      mask help: Place copyright information at the top of every subsystem in design.
      mask Display:
      | NxtrConf = 'Nexteer Confidential';
      | 
      | sys = bdroot; %handle for the current model ("system")
      | first = get_param(sys,'Created');
      | first = first(end-3:end);  %year is last four digits
      | 
      | last = get_param(sys,'LastModifiedDate');
      | if isempty(last)
      |     last = datestr(now,'yyyy');
      | else
      |     last = last(end-3:end);
      | end
      | 
      | if strcmp(first,last)
      |     fprintf('%s -- Copyright %s Nexteer',NxtrConf,first)
      | else
      |     fprintf('%s -- %s%s- %s Nexteer',NxtrConf,char(169),first,last)
      | end
  Ground : Ground
  RefTmr : Outport
  wires:
  Ground/1 -> RefTmr/1

== system CM660A_HwTq1Meas/HwTq1Meas/HwTq1MeasInit1/GetTiSpan1MicroSec32bit ==
  RefTmr : Inport
  CopyRight2 : Subsystem  Description=|  mask(Copyright Information){none=on}
      | Copyright info block.                                               
      |                                                                     
      | Place copyright information at the top of every subsystem in design.
      mask prompts: none "No parameters"
      mask help: Place copyright information at the top of every subsystem in design.
      mask Display:
      | NxtrConf = 'Nexteer Confidential';
      | 
      | sys = bdroot; %handle for the current model ("system")
      | first = get_param(sys,'Created');
      | first = first(end-3:end);  %year is last four digits
      | 
      | last = get_param(sys,'LastModifiedDate');
      | if isempty(last)
      |     last = datestr(now,'yyyy');
      | else
      |     last = last(end-3:end);
      | end
      | 
      | if strcmp(first,last)
      |     fprintf('%s -- Copyright %s Nexteer',NxtrConf,first)
      | else
      |     fprintf('%s -- %s%s- %s Nexteer',NxtrConf,char(169),first,last)
      | end
  Ground : Ground
  Terminator : Terminator
  TiSpan : Outport
  wires:
  Ground/1 -> TiSpan/1
  RefTmr/1 -> Terminator/1

== system CM660A_HwTq1Meas/HwTq1Meas/HwTq1MeasInit1/IoHwAb_SetFctPrphlHwTq1 ==
  CopyRight2 : Subsystem  Description=|  mask(Copyright Information){none=on}
      | Copyright info block.                                               
      |                                                                     
      | Place copyright information at the top of every subsystem in design.
      mask prompts: none "No parameters"
      mask help: Place copyright information at the top of every subsystem in design.
      mask Display:
      | NxtrConf = 'Nexteer Confidential';
      | 
      | sys = bdroot; %handle for the current model ("system")
      | first = get_param(sys,'Created');
      | first = first(end-3:end);  %year is last four digits
      | 
      | last = get_param(sys,'LastModifiedDate');
      | if isempty(last)
      |     last = datestr(now,'yyyy');
      | else
      |     last = last(end-3:end);
      | end
      | 
      | if strcmp(first,last)
      |     fprintf('%s -- Copyright %s Nexteer',NxtrConf,first)
      | else
      |     fprintf('%s -- %s%s- %s Nexteer',NxtrConf,char(169),first,last)
      | end

== system CM660A_HwTq1Meas/HwTq1Meas/HwTq1MeasPer1/CopyRight2 ==

== system CM660A_HwTq1Meas/HwTq1Meas/HwTq1MeasPer1/DebStepSelection ==
  TestOk : Inport
  CopyRight2 : Subsystem  Description=|  mask(Copyright Information){none=on}
      | Copyright info block.                                               
      |                                                                     
      | Place copyright information at the top of every subsystem in design.
      mask prompts: none "No parameters"
      mask help: Place copyright information at the top of every subsystem in design.
      mask Display:
      | NxtrConf = 'Nexteer Confidential';
      | 
      | sys = bdroot; %handle for the current model ("system")
      | first = get_param(sys,'Created');
      | first = first(end-3:end);  %year is last four digits
      | 
      | last = get_param(sys,'LastModifiedDate');
      | if isempty(last)
      |     last = datestr(now,'yyyy');
      | else
      |     last = last(end-3:end);
      | end
      | 
      | if strcmp(first,last)
      |     fprintf('%s -- Copyright %s Nexteer',NxtrConf,first)
      | else
      |     fprintf('%s -- %s%s- %s Nexteer',NxtrConf,char(169),first,last)
      | end
  NTCFailStepCal : Constant  Value=HwTq1MeasHwTq1PrtclFltFailStep  VectorParams1D=off
  NTCPassStepCal : Constant  Value=HwTq1MeasHwTq1PrtclFltPassStep
  Switch : Switch  Criteria=u2 > Threshold  Threshold=2
  DebStep : Outport
  wires:
  TestOk/1 -> Switch/2
  NTCPassStepCal/1 -> Switch/3
  Switch/1 -> DebStep/1
  NTCFailStepCal/1 -> Switch/1

== system CM660A_HwTq1Meas/HwTq1Meas/HwTq1MeasPer1/Do nothing ==
  Action Port : ActionPort
  CopyRight2 : Subsystem  Description=|  mask(Copyright Information){none=on}
      | Copyright info block.                                               
      |                                                                     
      | Place copyright information at the top of every subsystem in design.
      mask prompts: none "No parameters"
      mask help: Place copyright information at the top of every subsystem in design.
      mask Display:
      | NxtrConf = 'Nexteer Confidential';
      | 
      | sys = bdroot; %handle for the current model ("system")
      | first = get_param(sys,'Created');
      | first = first(end-3:end);  %year is last four digits
      | 
      | last = get_param(sys,'LastModifiedDate');
      | if isempty(last)
      |     last = datestr(now,'yyyy');
      | else
      |     last = last(end-3:end);
      | end
      | 
      | if strcmp(first,last)
      |     fprintf('%s -- Copyright %s Nexteer',NxtrConf,first)
      | else
      |     fprintf('%s -- %s%s- %s Nexteer',NxtrConf,char(169),first,last)
      | end

== system CM660A_HwTq1Meas/HwTq1Meas/HwTq1MeasPer1/GetNtcQlfr ==
  NtcNr : Inport
  CopyRight2 : Subsystem  Description=|  mask(Copyright Information){none=on}
      | Copyright info block.                                               
      |                                                                     
      | Place copyright information at the top of every subsystem in design.
      mask prompts: none "No parameters"
      mask help: Place copyright information at the top of every subsystem in design.
      mask Display:
      | NxtrConf = 'Nexteer Confidential';
      | 
      | sys = bdroot; %handle for the current model ("system")
      | first = get_param(sys,'Created');
      | first = first(end-3:end);  %year is last four digits
      | 
      | last = get_param(sys,'LastModifiedDate');
      | if isempty(last)
      |     last = datestr(now,'yyyy');
      | else
      |     last = last(end-3:end);
      | end
      | 
      | if strcmp(first,last)
      |     fprintf('%s -- Copyright %s Nexteer',NxtrConf,first)
      | else
      |     fprintf('%s -- %s%s- %s Nexteer',NxtrConf,char(169),first,last)
      | end
  Data Store Read : DataStoreRead  DataStoreName=Ntc0x075Qlfr
  Terminator : Terminator
  NtcQlfr : Outport
  wires:
  NtcNr/1 -> Terminator/1
  Data Store Read/1 -> NtcQlfr/1

== system CM660A_HwTq1Meas/HwTq1Meas/HwTq1MeasPer1/GetNtcQlfr1 ==
  NtcNr : Inport
  CopyRight2 : Subsystem  Description=|  mask(Copyright Information){none=on}
      | Copyright info block.                                               
      |                                                                     
      | Place copyright information at the top of every subsystem in design.
      mask prompts: none "No parameters"
      mask help: Place copyright information at the top of every subsystem in design.
      mask Display:
      | NxtrConf = 'Nexteer Confidential';
      | 
      | sys = bdroot; %handle for the current model ("system")
      | first = get_param(sys,'Created');
      | first = first(end-3:end);  %year is last four digits
      | 
      | last = get_param(sys,'LastModifiedDate');
      | if isempty(last)
      |     last = datestr(now,'yyyy');
      | else
      |     last = last(end-3:end);
      | end
      | 
      | if strcmp(first,last)
      |     fprintf('%s -- Copyright %s Nexteer',NxtrConf,first)
      | else
      |     fprintf('%s -- %s%s- %s Nexteer',NxtrConf,char(169),first,last)
      | end
  Data Store Read : DataStoreRead  DataStoreName=Ntc0x1E1Qlfr
  Terminator : Terminator
  NtcQlfr : Outport
  wires:
  NtcNr/1 -> Terminator/1
  Data Store Read/1 -> NtcQlfr/1

== system CM660A_HwTq1Meas/HwTq1Meas/HwTq1MeasPer1/HwTqCalculation ==
  RawHwTq : Inport
  CopyRight2 : Subsystem  Description=|  mask(Copyright Information){none=on}
      | Copyright info block.                                               
      |                                                                     
      | Place copyright information at the top of every subsystem in design.
      mask prompts: none "No parameters"
      mask help: Place copyright information at the top of every subsystem in design.
      mask Display:
      | NxtrConf = 'Nexteer Confidential';
      | 
      | sys = bdroot; %handle for the current model ("system")
      | first = get_param(sys,'Created');
      | first = first(end-3:end);  %year is last four digits
      | 
      | last = get_param(sys,'LastModifiedDate');
      | if isempty(last)
      |     last = datestr(now,'yyyy');
      | else
      |     last = last(end-3:end);
      | end
      | 
      | if strcmp(first,last)
      |     fprintf('%s -- Copyright %s Nexteer',NxtrConf,first)
      | else
      |     fprintf('%s -- %s%s- %s Nexteer',NxtrConf,char(169),first,last)
      | end
  Data Type Conversion : DataTypeConversion  OutDataTypeStr=single
  Data Type Conversion1 : DataTypeConversion  OutDataTypeStr=single
  HwTqOffs : Constant  Value=ELECGLBPRM_HWTQOFFS_HWNWTMTR_F32  OutDataTypeStr=single
  HwTqSca : Constant  Value=ELECGLBPRM_HWTQSCA_ULS_F32  OutDataTypeStr=single
  Product : Product
  Scope1 : Scope  NumInputPorts=2
      settings: YMin=-5~-5  YMax=5~5  SaveName=ScopeData2
  Substract : Sum  Inputs=+-
  HwTqData : Outport  OutDataTypeStr=single
  wires:
  HwTqSca/1 -> Product/2
  Product/1 -> Data Type Conversion1/1
  HwTqOffs/1 -> Substract/2
  Substract/1 -> Data Type Conversion/1
  RawHwTq/1 -> Product/1, Scope1/1
  Data Type Conversion1/1 -> Substract/1
  Data Type Conversion/1 -> Scope1/2, HwTqData/1

== system CM660A_HwTq1Meas/HwTq1Meas/HwTq1MeasPer1/If Action Subsystem1 ==
  Action Port : ActionPort  ActionType=then
  CopyRight2 : Subsystem  Description=|  mask(Copyright Information){none=on}
      | Copyright info block.                                               
      |                                                                     
      | Place copyright information at the top of every subsystem in design.
      mask prompts: none "No parameters"
      mask help: Place copyright information at the top of every subsystem in design.
      mask Display:
      | NxtrConf = 'Nexteer Confidential';
      | 
      | sys = bdroot; %handle for the current model ("system")
      | first = get_param(sys,'Created');
      | first = first(end-3:end);  %year is last four digits
      | 
      | last = get_param(sys,'LastModifiedDate');
      | if isempty(last)
      |     last = datestr(now,'yyyy');
      | else
      |     last = last(end-3:end);
      | end
      | 
      | if strcmp(first,last)
      |     fprintf('%s -- Copyright %s Nexteer',NxtrConf,first)
      | else
      |     fprintf('%s -- %s%s- %s Nexteer',NxtrConf,char(169),first,last)
      | end
  Data Type Conversion : DataTypeConversion  OutDataTypeStr=uint8
  SigQlfr : simulink/Sources/Enumerated Constant  OutDataTypeStr=Enum: SigQlfr1  Value=SigQlfr1.SIGQLFR_PASSD  SampleTime=inf
  Qlfr : Outport
  wires:
  SigQlfr/1 -> Data Type Conversion/1
  Data Type Conversion/1 -> Qlfr/1

== system CM660A_HwTq1Meas/HwTq1Meas/HwTq1MeasPer1/If Action Subsystem3 ==
  Action Port : ActionPort  ActionType=else
  CopyRight2 : Subsystem  Description=|  mask(Copyright Information){none=on}
      | Copyright info block.                                               
      |                                                                     
      | Place copyright information at the top of every subsystem in design.
      mask prompts: none "No parameters"
      mask help: Place copyright information at the top of every subsystem in design.
      mask Display:
      | NxtrConf = 'Nexteer Confidential';
      | 
      | sys = bdroot; %handle for the current model ("system")
      | first = get_param(sys,'Created');
      | first = first(end-3:end);  %year is last four digits
      | 
      | last = get_param(sys,'LastModifiedDate');
      | if isempty(last)
      |     last = datestr(now,'yyyy');
      | else
      |     last = last(end-3:end);
      | end
      | 
      | if strcmp(first,last)
      |     fprintf('%s -- Copyright %s Nexteer',NxtrConf,first)
      | else
      |     fprintf('%s -- %s%s- %s Nexteer',NxtrConf,char(169),first,last)
      | end
  Data Type Conversion : DataTypeConversion  OutDataTypeStr=uint8
  SigQlfr : simulink/Sources/Enumerated Constant  OutDataTypeStr=Enum: SigQlfr1  Value=SigQlfr1.SIGQLFR_FAILD  SampleTime=inf
  Qlfr : Outport
  wires:
  SigQlfr/1 -> Data Type Conversion/1
  Data Type Conversion/1 -> Qlfr/1

== system CM660A_HwTq1Meas/HwTq1Meas/HwTq1MeasPer1/PolarityEvaluation ==
  HwTqData : Inport  OutDataTypeStr=single
  HwTq1Polarity : Inport  RequirementInfo={} %GIDa_5e7beb6a_cd04_4438_bb0a_c4f4e2c14332  Port=2
  TestOk : Inport  Port=3
  CopyRight2 : Subsystem  Description=|  mask(Copyright Information){none=on}
      | Copyright info block.                                               
      |                                                                     
      | Place copyright information at the top of every subsystem in design.
      mask prompts: none "No parameters"
      mask help: Place copyright information at the top of every subsystem in design.
      mask Display:
      | NxtrConf = 'Nexteer Confidential';
      | 
      | sys = bdroot; %handle for the current model ("system")
      | first = get_param(sys,'Created');
      | first = first(end-3:end);  %year is last four digits
      | 
      | last = get_param(sys,'LastModifiedDate');
      | if isempty(last)
      |     last = datestr(now,'yyyy');
      | else
      |     last = last(end-3:end);
      | end
      | 
      | if strcmp(first,last)
      |     fprintf('%s -- Copyright %s Nexteer',NxtrConf,first)
      | else
      |     fprintf('%s -- %s%s- %s Nexteer',NxtrConf,char(169),first,last)
      | end
  Data Type Conversion : DataTypeConversion  OutDataTypeStr=single
  NVM Shadow RAM : DataStoreRead  DataStoreName=HwTq1OffsTrim
  PIM : DataStoreWrite  RequirementInfo={'doors' '00006115' '14' 'false' 'DOORS Surrogate Item' '' ; 'linktype_rmi_doors' '0000c47c (/ESG Group/FDD Module Requirements/EA4 Specific/CM660A_HwTq1Meas)' '#CM660A_50' 'true' 'REQ: CM660A_50' '' } %GIDa_077e43ec_662e_4d42_809b_03b059cade12  DataStoreName=HwTq1MeasPrevHwTq1
  PIM1 : DataStoreRead  DataStoreName=HwTq1MeasPrevHwTq1
  Product : Product  RequirementInfo={} %GIDa_582e6352_5967_4634_8e9a_a4093cfb2cb3
  Saturation : Saturate  UpperLimit=ELECGLBPRM_HWTQSATNUPPRLIM_HWNWTMTR_F32  LowerLimit=ELECGLBPRM_HWTQSATNLOWRLIM_HWNWTMTR_F32
  Subtract1 : Sum  Inputs=+-
  Switch : Switch  Criteria=u2 > Threshold  Threshold=2
  HwTq1 : Outport  RequirementInfo={'doors' '00006115' '15' 'false' 'DOORS Surrogate Item' '' ; 'linktype_rmi_doors' '0000c47c (/ESG Group/FDD Module Requirements/EA4 Specific/CM660A_HwTq1Meas)' '#CM660A_26' 'true' 'REQ: CM660A_26' '' } %GIDa_69c0e8a1_8bbe_4d59_a878_293d2bf0a501
  wires:
  Product/1 -> Switch/3
  TestOk/1 -> Switch/2
  Switch/1 -> PIM/1, Subtract1/1
  HwTq1Polarity/1 -> Data Type Conversion/1
  HwTqData/1 -> Product/1
  Data Type Conversion/1 -> Product/2
  Saturation/1 -> HwTq1/1
  Subtract1/1 -> Saturation/1
  NVM Shadow RAM/1 -> Subtract1/2
  PIM1/1 -> Switch/1

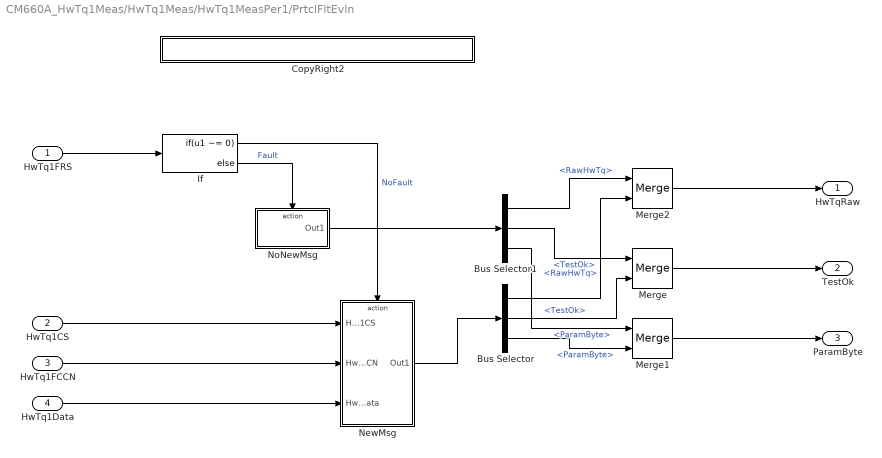
== system CM660A_HwTq1Meas/HwTq1Meas/HwTq1MeasPer1/PrtclFltEvln ==
  HwTq1FRS : Inport
  HwTq1CS : Inport  Port=2
  HwTq1FCCN : Inport  Port=3
  HwTq1Data : Inport  Port=4
  Bus Selector : BusSelector  OutputSignals=RawHwTq,TestOk,ParamByte
  Bus Selector1 : BusSelector  OutputSignals=RawHwTq,TestOk,ParamByte
  CopyRight2 : Subsystem  Description=|  mask(Copyright Information){none=on}
      | Copyright info block.                                               
      |                                                                     
      | Place copyright information at the top of every subsystem in design.
      mask prompts: none "No parameters"
      mask help: Place copyright information at the top of every subsystem in design.
      mask Display:
      | NxtrConf = 'Nexteer Confidential';
      | 
      | sys = bdroot; %handle for the current model ("system")
      | first = get_param(sys,'Created');
      | first = first(end-3:end);  %year is last four digits
      | 
      | last = get_param(sys,'LastModifiedDate');
      | if isempty(last)
      |     last = datestr(now,'yyyy');
      | else
      |     last = last(end-3:end);
      | end
      | 
      | if strcmp(first,last)
      |     fprintf('%s -- Copyright %s Nexteer',NxtrConf,first)
      | else
      |     fprintf('%s -- %s%s- %s Nexteer',NxtrConf,char(169),first,last)
      | end
  If : If  RequirementInfo={} %GIDa_27eddd86_3d73_4bbd_afc6_65cd0e917778  IfExpression=u1 ~= 0
  Merge : Merge
  Merge1 : Merge
  Merge2 : Merge
  NewMsg : Subsystem  RequirementInfo={'doors' '00006115' '17' 'false' 'DOORS Surrogate Item' '' } %GIDa_f428d820_7294_4433_be58_b2aad0418e6b  TreatAsAtomicUnit=on
      mask Display: disp('NewMsg')
  NoNewMsg : Subsystem  RequirementInfo={'doors' '00006115' '22' 'false' 'DOORS Surrogate Item' '' ; 'linktype_rmi_doors' '0000c47c (/ESG Group/FDD Module Requirements/EA4 Specific/CM660A_HwTq1Meas)' '#CM660A_47' 'true' 'REQ: CM660A_47' '' } %GIDa_9ee32e8d_1fd5_4b70_809d_63728be7576b  TreatAsAtomicUnit=on
      mask Display: disp('NoNewMsg')
  HwTqRaw : Outport
  TestOk : Outport  RequirementInfo={} %GIDa_95c6eb83_6b78_451b_a98a_b39fb65983b6  Port=2
  ParamByte : Outport  Port=3
  wires:
  HwTq1FRS/1 -> If/1
  If/1 -> NewMsg/Action  "NoFault"
  If/2 -> NoNewMsg/Action  "Fault"
  HwTq1CS/1 -> NewMsg/1(HwTq1CS)
  Merge/1 -> TestOk/1
  Merge1/1 -> ParamByte/1
  Merge2/1 -> HwTqRaw/1
  NewMsg/1(Out1) -> Bus Selector/1
  NoNewMsg/1(Out1) -> Bus Selector1/1
  Bus Selector1/1 -> Merge2/1  "<RawHwTq>"
  Bus Selector/1 -> Merge2/2  "<RawHwTq>"
  Bus Selector1/2 -> Merge/1  "<TestOk>"
  Bus Selector1/3 -> Merge1/1  "<ParamByte>"
  Bus Selector/2 -> Merge/2  "<TestOk>"
  Bus Selector/3 -> Merge1/2  "<ParamByte>"
  HwTq1FCCN/1 -> NewMsg/2(HwTq1FCCN)
  HwTq1Data/1 -> NewMsg/3(HwTq1Data)

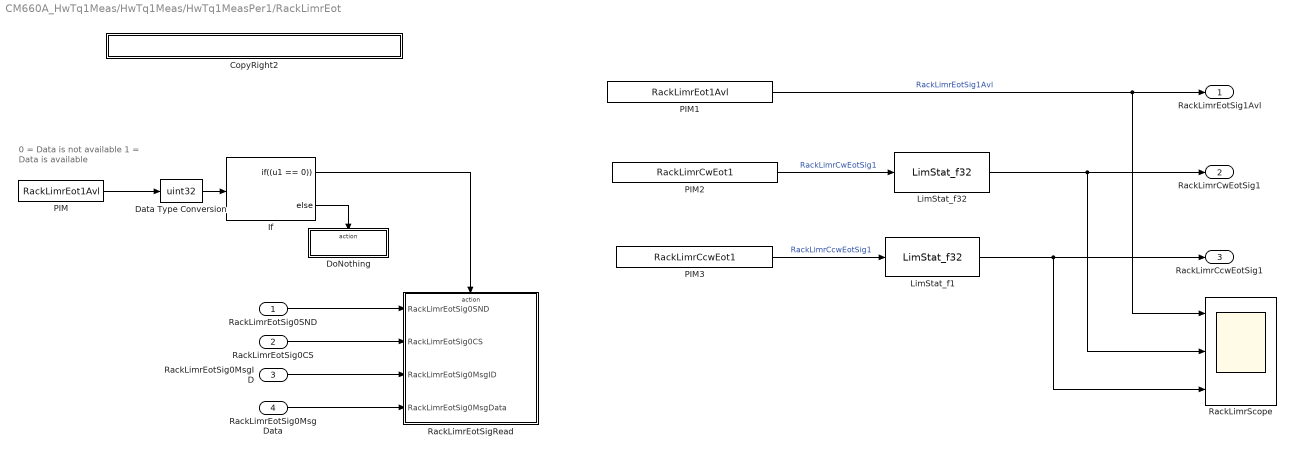
== system CM660A_HwTq1Meas/HwTq1Meas/HwTq1MeasPer1/RackLimrEot ==
  note: 0 = Data is not available
      | 1 = Data is available
  RackLimrEotSig0SND : Inport
  RackLimrEotSig0CS : Inport  Port=2
  RackLimrEotSig0MsgID : Inport  Port=3
  RackLimrEotSig0MsgData : Inport  Port=4
  CopyRight2 : Subsystem  Description=|  mask(Copyright Information){none=on}
      | Copyright info block.                                               
      |                                                                     
      | Place copyright information at the top of every subsystem in design.
      mask prompts: none "No parameters"
      mask help: Place copyright information at the top of every subsystem in design.
      mask Display:
      | NxtrConf = 'Nexteer Confidential';
      | 
      | sys = bdroot; %handle for the current model ("system")
      | first = get_param(sys,'Created');
      | first = first(end-3:end);  %year is last four digits
      | 
      | last = get_param(sys,'LastModifiedDate');
      | if isempty(last)
      |     last = datestr(now,'yyyy');
      | else
      |     last = last(end-3:end);
      | end
      | 
      | if strcmp(first,last)
      |     fprintf('%s -- Copyright %s Nexteer',NxtrConf,first)
      | else
      |     fprintf('%s -- %s%s- %s Nexteer',NxtrConf,char(169),first,last)
      | end
  Data Type Conversion : DataTypeConversion  OutDataTypeStr=uint32
  DoNothing : Subsystem  TreatAsAtomicUnit=on
  If : If  RequirementInfo={'linktype_rmi_doors' '0000c47c (/ESG Group/FDD Module Requirements/EA4 Specific/CM660A_HwTq1Meas)' '#CM660A_76' 'true' 'REQ: CM660A_76' '' } %GIDa_97ae3cdc_ee3b_4209_9f7f_e3776c69d98b  IfExpression=(u1 == 0)
  LimStat_f1 : NxtrLim/LimStat_f32  LoLim=RACKLIMREOTSIGLOLIM_HWDEG_F32  HiLim=0
      settings: AttributesFormatString=|
      | Low Limit: %<LoLim>
      | High Limit:%<HiLim>
  LimStat_f32 : NxtrLim/LimStat_f32  LoLim=0  HiLim=RACKLIMREOTSIGHILIM_HWDEG_F32
      settings: AttributesFormatString=|
      | Low Limit: %<LoLim>
      | High Limit:%<HiLim>
  PIM : DataStoreRead  DataStoreName=RackLimrEot1Avl
  PIM1 : DataStoreRead  RequirementInfo={'linktype_rmi_doors' '0000c47c (/ESG Group/FDD Module Requirements/EA4 Specific/CM660A_HwTq1Meas)' '#CM660A_75' 'true' 'REQ: CM660A_75' '' } %GIDa_392854b3_63b2_4906_80b7_a431b4afe123  DataStoreName=RackLimrEot1Avl
  PIM2 : DataStoreRead  RequirementInfo={'linktype_rmi_doors' '0000c47c (/ESG Group/FDD Module Requirements/EA4 Specific/CM660A_HwTq1Meas)' '#CM660A_70' 'true' 'REQ: CM660A_70' '' } %GIDa_17573b11_b989_4fbe_97c8_53900f7d59bd  DataStoreName=RackLimrCwEot1
  PIM3 : DataStoreRead  RequirementInfo={'linktype_rmi_doors' '0000c47c (/ESG Group/FDD Module Requirements/EA4 Specific/CM660A_HwTq1Meas)' '#CM660A_70' 'true' 'REQ: CM660A_70' '' } %GIDa_738d479f_26d5_4ed1_ad08_c0c77187e1ac  DataStoreName=RackLimrCcwEot1
  RackLimrEotSigRead : Subsystem  TreatAsAtomicUnit=on
  RackLimrScope : Scope  NumInputPorts=3
      settings: ShowLegends=on  TimeRange=20  YMin=-1~-100~-600  YMax=2~700~100
  RackLimrEotSig1Avl : Outport  RequirementInfo={} %GIDa_e207e200_0be5_4dbd_b5aa_9dcd133582ed
  RackLimrCwEotSig1 : Outport  RequirementInfo={} %GIDa_d68e745f_bbf7_4a55_9745_7febacfcaae5  Port=2
  RackLimrCcwEotSig1 : Outport  RequirementInfo={} %GIDa_d2e09d57_2587_426a_a7f5_ae8ec9b64963  Port=3
  wires:
  PIM/1 -> Data Type Conversion/1
  Data Type Conversion/1 -> If/1
  If/2 -> DoNothing/Action
  If/1 -> RackLimrEotSigRead/Action
  PIM2/1 -> LimStat_f32/1  "RackLimrCwEotSig1"
  PIM3/1 -> LimStat_f1/1  "RackLimrCcwEotSig1"
  PIM1/1 -> RackLimrScope/1, RackLimrEotSig1Avl/1  "RackLimrEotSig1Avl"
  LimStat_f32/1 -> RackLimrScope/2, RackLimrCwEotSig1/1
  LimStat_f1/1 -> RackLimrScope/3, RackLimrCcwEotSig1/1
  RackLimrEotSig0SND/1 -> RackLimrEotSigRead/1(RackLimrEotSig0SND)
  RackLimrEotSig0MsgID/1 -> RackLimrEotSigRead/3(RackLimrEotSig0MsgID)
  RackLimrEotSig0CS/1 -> RackLimrEotSigRead/2(RackLimrEotSig0CS)
  RackLimrEotSig0MsgData/1 -> RackLimrEotSigRead/4(RackLimrEotSig0MsgData)

== system CM660A_HwTq1Meas/HwTq1Meas/HwTq1MeasPer1/Read the Flag ==
  RegInpRSENT1FND : Inport
  Action Port : ActionPort
  CopyRight2 : Subsystem  Description=|  mask(Copyright Information){none=on}
      | Copyright info block.                                               
      |                                                                     
      | Place copyright information at the top of every subsystem in design.
      mask prompts: none "No parameters"
      mask help: Place copyright information at the top of every subsystem in design.
      mask Display:
      | NxtrConf = 'Nexteer Confidential';
      | 
      | sys = bdroot; %handle for the current model ("system")
      | first = get_param(sys,'Created');
      | first = first(end-3:end);  %year is last four digits
      | 
      | last = get_param(sys,'LastModifiedDate');
      | if isempty(last)
      |     last = datestr(now,'yyyy');
      | else
      |     last = last(end-3:end);
      | end
      | 
      | if strcmp(first,last)
      |     fprintf('%s -- Copyright %s Nexteer',NxtrConf,first)
      | else
      |     fprintf('%s -- %s%s- %s Nexteer',NxtrConf,char(169),first,last)
      | end
  RSENT1DummyRead : Terminator
  wires:
  RegInpRSENT1FND/1 -> RSENT1DummyRead/1

== system CM660A_HwTq1Meas/HwTq1Meas/HwTq1MeasPer1/SetNtcSts ==
  note: Note:
      |
      | - "ISO Fault Debounce Design" Simulink block intent to use here for Simulation purpose only. Do not Code this block
  NtcNr : Inport
  NtcStInfo : Inport  Port=2
  NtcSts : Inport  Port=3
  DebStep : Inport  Port=4
  CopyRight2 : Subsystem  Description=|  mask(Copyright Information){none=on}
      | Copyright info block.                                               
      |                                                                     
      | Place copyright information at the top of every subsystem in design.
      mask prompts: none "No parameters"
      mask help: Place copyright information at the top of every subsystem in design.
      mask Display:
      | NxtrConf = 'Nexteer Confidential';
      | 
      | sys = bdroot; %handle for the current model ("system")
      | first = get_param(sys,'Created');
      | first = first(end-3:end);  %year is last four digits
      | 
      | last = get_param(sys,'LastModifiedDate');
      | if isempty(last)
      |     last = datestr(now,'yyyy');
      | else
      |     last = last(end-3:end);
      | end
      | 
      | if strcmp(first,last)
      |     fprintf('%s -- Copyright %s Nexteer',NxtrConf,first)
      | else
      |     fprintf('%s -- %s%s- %s Nexteer',NxtrConf,char(169),first,last)
      | end
  Data Store Write : DataStoreWrite  DataStoreName=Ntc0x075Qlfr
  Ground : Ground
  ISO Fault Debounce Design : Stateflow chart  TreatAsAtomicUnit=on
      settings: AttributesFormatString=|
      | Simulation Purpose Only.
      | Do Not Code this block
      | Diagnostic Manager Owns this requirement
  Scope1 : Scope  NumInputPorts=3
      settings: YMin=-5~-5~-5  YMax=5~5~5  SaveName=ScopeData5
  Terminator : Terminator
  Terminator1 : Terminator
  wires:
  NtcStInfo/1 -> Terminator1/1
  NtcNr/1 -> Terminator/1
  NtcSts/1 -> ISO Fault Debounce Design/1(NtcSts), Scope1/1
  DebStep/1 -> ISO Fault Debounce Design/2(DebStep), Scope1/2
  ISO Fault Debounce Design/1(Qualifier) -> Scope1/3, Data Store Write/1
  Ground/1 -> ISO Fault Debounce Design/3(SvcClr)

== system CM660A_HwTq1Meas/HwTq1Meas/HwTq1MeasPer2/CopyRight2 ==

== system CM660A_HwTq1Meas/HwTq1Meas/HwTq1MeasPer2/If Action Subsystem ==
  Action Port : ActionPort  ActionType=then
  CopyRight2 : Subsystem  Description=|  mask(Copyright Information){none=on}
      | Copyright info block.                                               
      |                                                                     
      | Place copyright information at the top of every subsystem in design.
      mask prompts: none "No parameters"
      mask help: Place copyright information at the top of every subsystem in design.
      mask Display:
      | NxtrConf = 'Nexteer Confidential';
      | 
      | sys = bdroot; %handle for the current model ("system")
      | first = get_param(sys,'Created');
      | first = first(end-3:end);  %year is last four digits
      | 
      | last = get_param(sys,'LastModifiedDate');
      | if isempty(last)
      |     last = datestr(now,'yyyy');
      | else
      |     last = last(end-3:end);
      | end
      | 
      | if strcmp(first,last)
      |     fprintf('%s -- Copyright %s Nexteer',NxtrConf,first)
      | else
      |     fprintf('%s -- %s%s- %s Nexteer',NxtrConf,char(169),first,last)
      | end
  Data Type Conversion : DataTypeConversion  OutDataTypeStr=uint8
  NoFlt : Constant  RequirementInfo={} %GIDa_73f0a11e_cf31_48e6_8bb2_3cf4b1949e36  Value=ELECGLBPRM_NOFLT_CNT_U08  OutDataTypeStr=uint8
  NtcSts : simulink/Sources/Enumerated Constant  OutDataTypeStr=Enum: NtcSts1  Value=NtcSts1.NTCSTS_PASSD  SampleTime=inf
  ParamByte : Outport
  TestOk : Outport  Port=2
  wires:
  NtcSts/1 -> Data Type Conversion/1
  NoFlt/1 -> ParamByte/1
  Data Type Conversion/1 -> TestOk/1

== system CM660A_HwTq1Meas/HwTq1Meas/HwTq1MeasPer2/If Action Subsystem1 ==
  Action Port : ActionPort  ActionType=else
  CopyRight2 : Subsystem  Description=|  mask(Copyright Information){none=on}
      | Copyright info block.                                               
      |                                                                     
      | Place copyright information at the top of every subsystem in design.
      mask prompts: none "No parameters"
      mask help: Place copyright information at the top of every subsystem in design.
      mask Display:
      | NxtrConf = 'Nexteer Confidential';
      | 
      | sys = bdroot; %handle for the current model ("system")
      | first = get_param(sys,'Created');
      | first = first(end-3:end);  %year is last four digits
      | 
      | last = get_param(sys,'LastModifiedDate');
      | if isempty(last)
      |     last = datestr(now,'yyyy');
      | else
      |     last = last(end-3:end);
      | end
      | 
      | if strcmp(first,last)
      |     fprintf('%s -- Copyright %s Nexteer',NxtrConf,first)
      | else
      |     fprintf('%s -- %s%s- %s Nexteer',NxtrConf,char(169),first,last)
      | end
  Data Type Conversion : DataTypeConversion  OutDataTypeStr=uint8
  NoFlt : Constant  RequirementInfo={} %GIDa_eae82ea4_69e1_4b6f_94ef_18d1f1394a46  Value=ELECGLBPRM_OFFSTRIMNOTPRFM_CNT_U08  OutDataTypeStr=uint8
  NtcSts : simulink/Sources/Enumerated Constant  OutDataTypeStr=Enum: NtcSts1  Value=NtcSts1.NTCSTS_FAILD  SampleTime=inf
  ParamByte : Outport
  TestOk : Outport  Port=2
  wires:
  NoFlt/1 -> ParamByte/1
  NtcSts/1 -> Data Type Conversion/1
  Data Type Conversion/1 -> TestOk/1

== system CM660A_HwTq1Meas/HwTq1Meas/HwTq1MeasPer2/SetNtcSts ==
  note: Note:
      |
      | - "ISO Fault Debounce Design" Simulink block intent to use here for Simulation purpose only. Do not Code this block
  NtcNr : Inport
  NtcStInfo : Inport  Port=2
  NtcSts : Inport  Port=3
  DebStep : Inport  Port=4
  CopyRight2 : Subsystem  Description=|  mask(Copyright Information){none=on}
      | Copyright info block.                                               
      |                                                                     
      | Place copyright information at the top of every subsystem in design.
      mask prompts: none "No parameters"
      mask help: Place copyright information at the top of every subsystem in design.
      mask Display:
      | NxtrConf = 'Nexteer Confidential';
      | 
      | sys = bdroot; %handle for the current model ("system")
      | first = get_param(sys,'Created');
      | first = first(end-3:end);  %year is last four digits
      | 
      | last = get_param(sys,'LastModifiedDate');
      | if isempty(last)
      |     last = datestr(now,'yyyy');
      | else
      |     last = last(end-3:end);
      | end
      | 
      | if strcmp(first,last)
      |     fprintf('%s -- Copyright %s Nexteer',NxtrConf,first)
      | else
      |     fprintf('%s -- %s%s- %s Nexteer',NxtrConf,char(169),first,last)
      | end
  Data Store Write : DataStoreWrite  DataStoreName=Ntc0x1E1Qlfr
  Ground : Ground
  ISO Fault Debounce Design : Stateflow chart  TreatAsAtomicUnit=on
      settings: AttributesFormatString=|
      | Simulation Purpose Only.
      | Do Not Code this block
      | Diagnostic Manager Owns this requirement
  Scope1 : Scope  NumInputPorts=3
      settings: YMin=-5~-5~-5  YMax=5~5~5  SaveName=ScopeData5
  Terminator : Terminator
  Terminator1 : Terminator
  wires:
  Ground/1 -> ISO Fault Debounce Design/3(SvcClr)
  ISO Fault Debounce Design/1(Qualifier) -> Data Store Write/1, Scope1/3
  DebStep/1 -> Scope1/2, ISO Fault Debounce Design/2(DebStep)
  NtcSts/1 -> Scope1/1, ISO Fault Debounce Design/1(NtcSts)
  NtcNr/1 -> Terminator/1
  NtcStInfo/1 -> Terminator1/1

== system CM660A_HwTq1Meas/HwTq1Meas/HwTq1MeasTrigStrt/CopyRight2 ==

== system CM660A_HwTq1Meas/HwTq1Meas/HwTq1MeasTrigStrt/GetRefTmr1MicroSec32bit ==
  CopyRight2 : Subsystem  Description=|  mask(Copyright Information){none=on}
      | Copyright info block.                                               
      |                                                                     
      | Place copyright information at the top of every subsystem in design.
      mask prompts: none "No parameters"
      mask help: Place copyright information at the top of every subsystem in design.
      mask Display:
      | NxtrConf = 'Nexteer Confidential';
      | 
      | sys = bdroot; %handle for the current model ("system")
      | first = get_param(sys,'Created');
      | first = first(end-3:end);  %year is last four digits
      | 
      | last = get_param(sys,'LastModifiedDate');
      | if isempty(last)
      |     last = datestr(now,'yyyy');
      | else
      |     last = last(end-3:end);
      | end
      | 
      | if strcmp(first,last)
      |     fprintf('%s -- Copyright %s Nexteer',NxtrConf,first)
      | else
      |     fprintf('%s -- %s%s- %s Nexteer',NxtrConf,char(169),first,last)
      | end
  Ground : Ground
  RefTmr : Outport
  wires:
  Ground/1 -> RefTmr/1

== system CM660A_HwTq1Meas/HwTq1Meas/HwTq1MeasTrigStrt/GetTiSpan1MicroSec32bit ==
  RefTmr : Inport
  CopyRight2 : Subsystem  Description=|  mask(Copyright Information){none=on}
      | Copyright info block.                                               
      |                                                                     
      | Place copyright information at the top of every subsystem in design.
      mask prompts: none "No parameters"
      mask help: Place copyright information at the top of every subsystem in design.
      mask Display:
      | NxtrConf = 'Nexteer Confidential';
      | 
      | sys = bdroot; %handle for the current model ("system")
      | first = get_param(sys,'Created');
      | first = first(end-3:end);  %year is last four digits
      | 
      | last = get_param(sys,'LastModifiedDate');
      | if isempty(last)
      |     last = datestr(now,'yyyy');
      | else
      |     last = last(end-3:end);
      | end
      | 
      | if strcmp(first,last)
      |     fprintf('%s -- Copyright %s Nexteer',NxtrConf,first)
      | else
      |     fprintf('%s -- %s%s- %s Nexteer',NxtrConf,char(169),first,last)
      | end
  Ground : Ground
  Terminator : Terminator
  TiSpan : Outport
  wires:
  RefTmr/1 -> Terminator/1
  Ground/1 -> TiSpan/1

== system CM660A_HwTq1Meas/HwTq1Meas/HwTq1MeasInit1/GetRefTmr1MicroSec32bit/CopyRight2 ==

== system CM660A_HwTq1Meas/HwTq1Meas/HwTq1MeasInit1/GetTiSpan1MicroSec32bit/CopyRight2 ==

== system CM660A_HwTq1Meas/HwTq1Meas/HwTq1MeasInit1/IoHwAb_SetFctPrphlHwTq1/CopyRight2 ==

== system CM660A_HwTq1Meas/HwTq1Meas/HwTq1MeasPer1/DebStepSelection/CopyRight2 ==

== system CM660A_HwTq1Meas/HwTq1Meas/HwTq1MeasPer1/Do nothing/CopyRight2 ==

== system CM660A_HwTq1Meas/HwTq1Meas/HwTq1MeasPer1/GetNtcQlfr/CopyRight2 ==

== system CM660A_HwTq1Meas/HwTq1Meas/HwTq1MeasPer1/GetNtcQlfr1/CopyRight2 ==

== system CM660A_HwTq1Meas/HwTq1Meas/HwTq1MeasPer1/HwTqCalculation/CopyRight2 ==

== system CM660A_HwTq1Meas/HwTq1Meas/HwTq1MeasPer1/If Action Subsystem1/CopyRight2 ==

== system CM660A_HwTq1Meas/HwTq1Meas/HwTq1MeasPer1/If Action Subsystem3/CopyRight2 ==

== system CM660A_HwTq1Meas/HwTq1Meas/HwTq1MeasPer1/PolarityEvaluation/CopyRight2 ==

== system CM660A_HwTq1Meas/HwTq1Meas/HwTq1MeasPer1/PrtclFltEvln/CopyRight2 ==

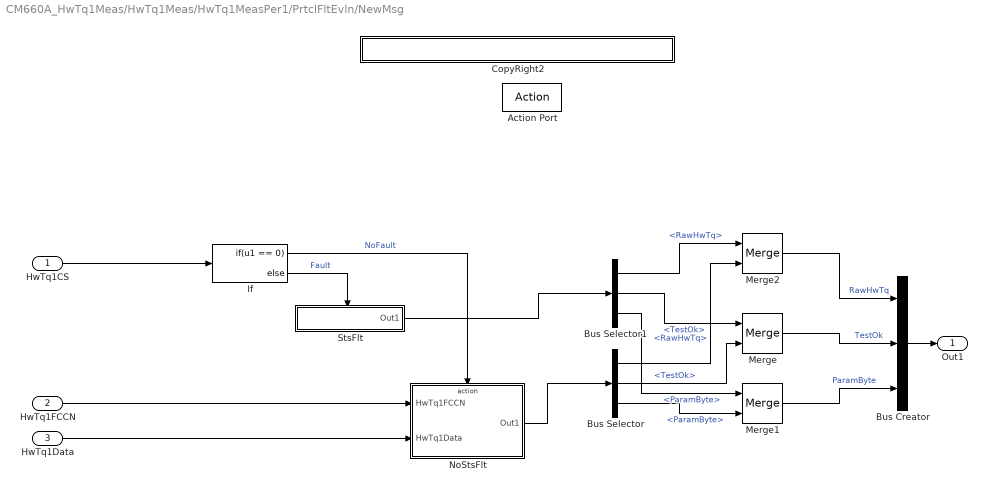
== system CM660A_HwTq1Meas/HwTq1Meas/HwTq1MeasPer1/PrtclFltEvln/NewMsg ==
  HwTq1CS : Inport
  HwTq1FCCN : Inport  Port=2
  HwTq1Data : Inport  Port=3
  Action Port : ActionPort  ActionType=then
  Bus Creator : BusCreator  Inputs=3
  Bus Selector : BusSelector  OutputSignals=RawHwTq,TestOk,ParamByte
  Bus Selector1 : BusSelector  OutputSignals=RawHwTq,TestOk,ParamByte
  CopyRight2 : Subsystem  Description=|  mask(Copyright Information){none=on}
      | Copyright info block.                                               
      |                                                                     
      | Place copyright information at the top of every subsystem in design.
      mask prompts: none "No parameters"
      mask help: Place copyright information at the top of every subsystem in design.
      mask Display:
      | NxtrConf = 'Nexteer Confidential';
      | 
      | sys = bdroot; %handle for the current model ("system")
      | first = get_param(sys,'Created');
      | first = first(end-3:end);  %year is last four digits
      | 
      | last = get_param(sys,'LastModifiedDate');
      | if isempty(last)
      |     last = datestr(now,'yyyy');
      | else
      |     last = last(end-3:end);
      | end
      | 
      | if strcmp(first,last)
      |     fprintf('%s -- Copyright %s Nexteer',NxtrConf,first)
      | else
      |     fprintf('%s -- %s%s- %s Nexteer',NxtrConf,char(169),first,last)
      | end
  If : If  IfExpression=u1 == 0
  Merge : Merge
  Merge1 : Merge
  Merge2 : Merge
  NoStsFlt : Subsystem  RequirementInfo={'doors' '00006115' '18' 'false' 'DOORS Surrogate Item' '' } %GIDa_ac6611b7_c860_4920_977e_a7e9bf2750f4  TreatAsAtomicUnit=on
  StsFlt : Subsystem  RequirementInfo={'doors' '00006115' '21' 'false' 'DOORS Surrogate Item' '' ; 'linktype_rmi_doors' '0000c47c (/ESG Group/FDD Module Requirements/EA4 Specific/CM660A_HwTq1Meas)' '#CM660A_40' 'true' 'REQ: CM660A_40' '' ; 'linktype_rmi_doors' '0000c47c (/ESG Group/FDD Module Requirements/EA4 Specific/CM660A_HwTq1Meas)' '#CM660A_41' 'true' 'REQ: CM660A_41' '' ; 'linktype_rmi_doors' '0000c47c (/ESG Group/FDD Module Requirements/EA4 Specific/CM660A_HwTq1Meas)' '#CM660A_42' 'true' 'REQ: CM660A_42' '' ; 'linktype_rmi_doors' '0000c47c (/ESG Group/FDD Module Requirements/EA4 Specific/CM660A_HwTq1Meas)' '#CM660A_43' 'true' 'REQ: CM660A_43' '' ; 'linktype_rmi_doors' '0000c47c (/ESG Group/FDD Module Requirements/EA4 Specific/CM660A_HwTq1Meas)' '#CM660A_44' 'true' 'REQ: CM660A_44' '' ; 'linktype_rmi_doors' '0000c47c (/ESG Group/FDD Module Requirements/EA4 Specific/CM660A_HwTq1Meas)' '#CM660A_45' 'true' 'REQ: CM660A_45' '' ; 'linktype_rmi_doors' '0000c47c (/ESG Group/FDD Module Requirements/EA4 Specific/CM660A_HwTq1Meas)' '#CM660A_46' 'true' 'REQ: CM660A_46' '' } %GIDa_679ffcb4_3849_4021_9957_65733ff452c6  TreatAsAtomicUnit=on
      mask Display: disp('STSFLT')
  Out1 : Outport
  wires:
  If/1 -> NoStsFlt/Action  "NoFault"
  If/2 -> StsFlt/Action  "Fault"
  Merge/1 -> Bus Creator/2  "TestOk"
  Merge1/1 -> Bus Creator/3  "ParamByte"
  Merge2/1 -> Bus Creator/1  "RawHwTq"
  NoStsFlt/1(Out1) -> Bus Selector/1
  StsFlt/1(Out1) -> Bus Selector1/1
  Bus Selector1/1 -> Merge2/1  "<RawHwTq>"
  Bus Selector/1 -> Merge2/2  "<RawHwTq>"
  Bus Selector1/2 -> Merge/1  "<TestOk>"
  Bus Selector1/3 -> Merge1/1  "<ParamByte>"
  Bus Selector/2 -> Merge/2  "<TestOk>"
  Bus Selector/3 -> Merge1/2  "<ParamByte>"
  Bus Creator/1 -> Out1/1
  HwTq1CS/1 -> If/1
  HwTq1FCCN/1 -> NoStsFlt/1(HwTq1FCCN)
  HwTq1Data/1 -> NoStsFlt/2(HwTq1Data)

== system CM660A_HwTq1Meas/HwTq1Meas/HwTq1MeasPer1/PrtclFltEvln/NoNewMsg ==
  Action Port : ActionPort  ActionType=else
  Add : Sum
  Bus Creator : BusCreator  Inputs=3
  Constant1 : Constant  OutDataTypeStr=uint32
  CopyRight2 : Subsystem  Description=|  mask(Copyright Information){none=on}
      | Copyright info block.                                               
      |                                                                     
      | Place copyright information at the top of every subsystem in design.
      mask prompts: none "No parameters"
      mask help: Place copyright information at the top of every subsystem in design.
      mask Display:
      | NxtrConf = 'Nexteer Confidential';
      | 
      | sys = bdroot; %handle for the current model ("system")
      | first = get_param(sys,'Created');
      | first = first(end-3:end);  %year is last four digits
      | 
      | last = get_param(sys,'LastModifiedDate');
      | if isempty(last)
      |     last = datestr(now,'yyyy');
      | else
      |     last = last(end-3:end);
      | end
      | 
      | if strcmp(first,last)
      |     fprintf('%s -- Copyright %s Nexteer',NxtrConf,first)
      | else
      |     fprintf('%s -- %s%s- %s Nexteer',NxtrConf,char(169),first,last)
      | end
  Data Type Conversion : DataTypeConversion  OutDataTypeStr=uint8
  NtcSts : simulink/Sources/Enumerated Constant  OutDataTypeStr=Enum: NtcSts1  Value=NtcSts1.NTCSTS_PREFAILD  SampleTime=inf
  PIM : DataStoreWrite  RequirementInfo={} %GIDa_d7aaed20_af5c_45d0_a82c_a669b9da5dc5  DataStoreName=HwTq1MsgMissRxCnt
  PIM1 : DataStoreRead  DataStoreName=HwTq1MsgMissRxCnt
  PRTCL_FAULT : Constant  Value=ELECGLBPRM_PRTCLFLT_CNT_U08  OutDataTypeStr=uint8
  Signal Conversion : SignalConversion
  Trq : Constant  Value=0  OutDataTypeStr=uint32
  Out1 : Outport
  wires:
  NtcSts/1 -> Data Type Conversion/1
  PRTCL_FAULT/1 -> Bus Creator/3  "ParamByte"
  Data Type Conversion/1 -> Bus Creator/2  "TestOk"
  Trq/1 -> Bus Creator/1  "RawHwTq"
  Bus Creator/1 -> Signal Conversion/1
  Signal Conversion/1 -> Out1/1
  Add/1 -> PIM/1
  Constant1/1 -> Add/2
  PIM1/1 -> Add/1

== system CM660A_HwTq1Meas/HwTq1Meas/HwTq1MeasPer1/RackLimrEot/CopyRight2 ==
